simulink model "souk_dual_pipeline_krm"  (R2021a)
settings: Solver=VariableStepAuto  StartTime=0.0  StopTime=10.0  RelTol=1e-3
undefined symbols (not defined in the file): datetime, emio_enet2_tsu_timer_cmp_val_0, posixtime, signal
libraries: xbsIndex_r4 x15746, casper_library_misc x108, casper_library_delays x65, casper_library_reorder x44, xps_library x12
(part 3 of 175)

== system souk_dual_pipeline_krm/KRM4ZUxx ==

== system souk_dual_pipeline_krm/bus_expand ==
  bus_in : Inport
  reinterpret1 : xbsIndex_r4/Reinterpret  force_arith_type=on  arith_type=Unsigned  force_bin_pt=on  bin_pt=0  block_type=reinterpret
  reinterpret2 : xbsIndex_r4/Reinterpret  force_arith_type=on  arith_type=Unsigned  force_bin_pt=on  bin_pt=0  block_type=reinterpret
  slice1 : xbsIndex_r4/Slice  nbits=256  boolean_output=off  mode=Upper Bit Location + Width  bit1=-256  base1=MSB of Input  bit0=0  base0=LSB of Input  dbl_ovrd=off  block_type=slice
  slice2 : xbsIndex_r4/Slice  nbits=256  boolean_output=off  mode=Upper Bit Location + Width  bit1=0  base1=MSB of Input  bit0=0  base0=LSB of Input  dbl_ovrd=off  block_type=slice
  msb_out2 : Outport  VectorParamsAs1DForOutWhenUnconnected=off
  lsb_out1 : Outport  Port=2  VectorParamsAs1DForOutWhenUnconnected=off
  wires:
  bus_in/1 -> slice2/1, slice1/1
  slice2/1 -> reinterpret2/1
  reinterpret2/1 -> msb_out2/1
  slice1/1 -> reinterpret1/1
  reinterpret1/1 -> lsb_out1/1

== system souk_dual_pipeline_krm/bus_expand1 ==
  bus_in : Inport
  reinterpret1 : xbsIndex_r4/Reinterpret  force_arith_type=on  arith_type=Unsigned  force_bin_pt=on  bin_pt=0  block_type=reinterpret
  reinterpret2 : xbsIndex_r4/Reinterpret  force_arith_type=on  arith_type=Unsigned  force_bin_pt=on  bin_pt=0  block_type=reinterpret
  slice1 : xbsIndex_r4/Slice  nbits=256  boolean_output=off  mode=Upper Bit Location + Width  bit1=-256  base1=MSB of Input  bit0=0  base0=LSB of Input  dbl_ovrd=off  block_type=slice
  slice2 : xbsIndex_r4/Slice  nbits=256  boolean_output=off  mode=Upper Bit Location + Width  bit1=0  base1=MSB of Input  bit0=0  base0=LSB of Input  dbl_ovrd=off  block_type=slice
  msb_out2 : Outport  VectorParamsAs1DForOutWhenUnconnected=off
  lsb_out1 : Outport  Port=2  VectorParamsAs1DForOutWhenUnconnected=off
  wires:
  reinterpret1/1 -> lsb_out1/1
  slice1/1 -> reinterpret1/1
  reinterpret2/1 -> msb_out2/1
  slice2/1 -> reinterpret2/1
  bus_in/1 -> slice1/1, slice2/1

== system souk_dual_pipeline_krm/common ==
  note: flip channels and
      | put first sample in MSB
  autocorr_sync0 : Inport
  autocorr_din0 : Inport  Port=2
  autocorr_rst0 : Inport  Port=3
  autocorr_sync1 : Inport  Port=4
  autocorr_din1 : Inport  Port=5
  autocorr_rst1 : Inport  Port=6
  autocorr_sync2 : Inport  Port=7
  autocorr_din2 : Inport  Port=8
  autocorr_rst2 : Inport  Port=9
  autocorr_sync3 : Inport  Port=10
  autocorr_din3 : Inport  Port=11
  autocorr_rst3 : Inport  Port=12
  input0 : Inport  Port=13
  input1 : Inport  Port=14
  input2 : Inport  Port=15
  input3 : Inport  Port=16
  output0 : Inport  Port=17
  output1 : Inport  Port=18
  output2 : Inport  Port=19
  output3 : Inport  Port=20
  tt0 : Inport  Port=21
  tt1 : Inport  Port=22
  tt2 : Inport  Port=23
  tt3 : Inport  Port=24
  Delay{,1..29} (30 alike) : xbsIndex_r4/Delay  rst=off  infoeditControl=Selection of Reset will increase slice count due to use of real FFs and instead of SRLs  en=off  latency=1  reg_retiming=off  dbl_ovrd=off  block_type=delay
  Mux{,1..5} (6 alike) : xbsIndex_r4/Mux  inputs=4  en=off  latency=1  precision=Full  arith_type=Unsigned  n_bits=16  bin_pt=14  quantization=Truncate  overflow=Wrap  dbl_ovrd=off  block_type=mux
  adc_ss : Subsystem  mask{ram_depth_bits=9}
      mask prompts: ram_depth_bits "Ram depth (2^?)"
  autocorr : Subsystem  mask{nchan_bits=13-4, npol_bits=0}
      mask prompts: nchan_bits "Number of *SERIAL* channels (2^?)"; npol_bits "Number of pols (2^?)"
  bus_expand : Subsystem  AncestorBlock=casper_library_flow_control/bus_expand  mask(bus_expand){mode=divisions of equal size, outputNum=2, outputWidth=16*8, outputBinaryPt=0, outputArithmeticType=0, show_format=off, outputToWorkspace=off, variablePrefix=out, outputToModelAsWell=on}
      mask prompts: outputNum "Number of outputs:"; outputWidth "Output width:"; outputBinaryPt "Output binary point position:"; outputArithmeticType "Output arithmetic type (ufix=0, fix=1, bool=2):"; show_format "Print format string?"; outputToWorkspace "Output to workspace?"; variablePrefix "Variable name prefix:"; outputToModelAsWell "Output to model as well?"
      mask help:
      | Expands a 'bus' made using a bus_create or Xilinx
      | concat block.
      | The input will be divided into the specified number
      | of outputs with the specified arithmetic types.
      | Divisions are made from most significant bit.
      mask init: same as souk_dual_pipeline_krm/bus_expand
      settings: AttributesFormatString=2 outputs
      mask TypeOptions mode: divisions of equal size | divisions of arbitrary size
      mask Callback mode: %bus_expand_callback();
      mask Callback outputWidth: %bus_expand_callback();
      mask Callback outputToWorkspace: %bus_expand_callback();
  bus_expand1 : Subsystem  AncestorBlock=casper_library_flow_control/bus_expand  mask(bus_expand){mode=divisions of equal size, outputNum=2, outputWidth=16*16, outputBinaryPt=0, outputArithmeticType=0, show_format=off, outputToWorkspace=off, variablePrefix=out, outputToModelAsWell=on}
      mask prompts: outputNum "Number of outputs:"; outputWidth "Output width:"; outputBinaryPt "Output binary point position:"; outputArithmeticType "Output arithmetic type (ufix=0, fix=1, bool=2):"; show_format "Print format string?"; outputToWorkspace "Output to workspace?"; variablePrefix "Variable name prefix:"; outputToModelAsWell "Output to model as well?"
      mask help:
      | Expands a 'bus' made using a bus_create or Xilinx
      | concat block.
      | The input will be divided into the specified number
      | of outputs with the specified arithmetic types.
      | Divisions are made from most significant bit.
      mask init: same as souk_dual_pipeline_krm/bus_expand
      settings: AttributesFormatString=2 outputs
      mask TypeOptions mode: divisions of equal size | divisions of arbitrary size
      mask Callback mode: %bus_expand_callback();
      mask Callback outputWidth: %bus_expand_callback();
      mask Callback outputToWorkspace: %bus_expand_callback();
  cordic_gen : Subsystem  mask{n_cordic=1, n_parallel=8}
      mask prompts: n_cordic "Number of independent generators?"; n_parallel "Number of parallel samples?"
  dac_ss : Subsystem  mask{ram_depth_bits=9}
      mask prompts: ram_depth_bits "Ram depth (2^?)"
  iq_deinterleave : Subsystem  AncestorBlock=casper_library_flow_control/munge  mask(munge){divisions=16, div_size=16*ones(16,1), order=reshape(transpose(reshape([0:15], [2,8])), [16,1]), arith_type_out=Unsigned, bin_pt_out=0}
      mask prompts: divisions "Number of divisions"; div_size "Division size (bits)"; order "Division packing order"; arith_type_out "Output arithmetic type"; bin_pt_out "Output binary point"
      mask help: Splits an input bus into the specified number of divisions and then recombines them in the order specified (most significant division = 0,least = number divisions-1)
      mask init:
      | munge_init(gcb, ...
      |     'divisions', divisions, ...
      |     'div_size', div_size, ...
      |     'order', order, ...
      |     'arith_type_out', arith_type_out, ...
      |     'bin_pt_out', bin_pt_out);
      settings: AttributesFormatString=|
      | split:[16;16;16;16;16;16;16;16;16;16;16;16;16;16;16;16]
      | join:[0;2;4;6;8;10;12;14;1;3;5;7;9;11;13;15]
      | Unsigned [256,0]
      mask TypeOptions arith_type_out: Unsigned | Signed  (2's comp) | Floating-point
  lut_gen : Subsystem  mask{n_generator=1, n_parallel=8, n_sample_bits=13}
      mask prompts: n_generator "Number of independent generators?"; n_parallel "Number of parallel samples?"; n_sample_bits "Number of samples total (2^?)"
  munge : Subsystem  AncestorBlock=casper_library_flow_control/munge  mask(munge){divisions=32, div_size=16*ones(32,1), order=[31:-1:0], arith_type_out=Unsigned, bin_pt_out=0}
      mask prompts: divisions "Number of divisions"; div_size "Division size (bits)"; order "Division packing order"; arith_type_out "Output arithmetic type"; bin_pt_out "Output binary point"
      mask help: Splits an input bus into the specified number of divisions and then recombines them in the order specified (most significant division = 0,least = number divisions-1)
      mask init:
      | munge_init(gcb, ...
      |     'divisions', divisions, ...
      |     'div_size', div_size, ...
      |     'order', order, ...
      |     'arith_type_out', arith_type_out, ...
      |     'bin_pt_out', bin_pt_out);
      settings: AttributesFormatString=|
      | split:[16;16;16;16;16;16;16;16;16;16;16;16;16;16;16;16;16;16;16;16;16;16;16;16;16;16;16;16;16;16;16;16]
      | join:[31 30 29 28 27 26 25 24 23 22 21 20 19 18 17 16 15 14 13 12 11 10 9 8 7 6 5 4 3 2 1 0]
      | Unsigned [512,0]
      mask TypeOptions arith_type_out: Unsigned | Signed  (2's comp) | Floating-point
  sel : Subsystem  Tag=xps:sw_reg  AncestorBlock=xps_library/Memory/software_register  mask(swreg){io_dir=From Processor, io_delay=0, init_val=dec2hex(0), sample_period=1, names=reg, bitwidths=2, bin_pts=0, arith_types=0, sim_port=on, show_format=on, desc_str=""}
      mask prompts: io_dir "I/O direction"; io_delay "I/O delay"; init_val "Initial Value"; sample_period "Sample period"; names "Bitfield names [msb...lsb]"; bitwidths "Bitfield widths"; bin_pts "Bitfield binary pts"; arith_types "Bitfield types, ufix=0, fix=1, bool=2"; sim_port "Provide sim input/output?"; show_format "Print format string?"; desc_str "Description"
      mask help: A 32-bit software-accessible register. Can be divided into bitfields of varying widths and types using the fields in the block mask.
      mask init:
      | swreg_init(gcb)
      settings: AttributesFormatString=1input:uf2.0 = 2 bits
      mask TypeOptions io_dir: To Processor | From Processor
      mask Callback io_dir:
      | mask_enables = get_param(gcb, 'MaskEnables');
      | mask_names = get_param(gcb, 'MaskNames');
      | if strcmp(get_param(gcb, 'io_dir'), 'To Processor'),
      |     mask_enables{ismember(mask_names, 'sample_period')} = 'off';
      | else
      |     mask_enables{ismember(mask_names, 'sample_period')} = 'on';
      | end
      | set_param(gcb, 'MaskEnables', mask_enables);
      mask DialogControl ParameterTabVar0 Prompt: Setup
  zoom_acc : Subsystem  mask{nchan_serial_bits=10, downsample_factor=512}
      mask prompts: nchan_serial_bits "Number of serial channels (2^?)"; downsample_factor "Downsample factor?"
  zoom_fft : Subsystem
  cordic_gen_out : Outport
  lut_gen_out : Outport  Port=2
  wires:
  lut_gen/1(dout) -> lut_gen_out/1
  cordic_gen/1(dout) -> cordic_gen_out/1
  autocorr_sync0/1 -> Delay6/1
  autocorr_sync1/1 -> Delay7/1
  Delay/1 -> Mux/1
  Delay1/1 -> Mux1/1
  Delay2/1 -> Mux2/1
  zoom_fft/1(sync_out) -> zoom_acc/1(sync)
  zoom_fft/2(dout) -> zoom_acc/2(din)
  Mux2/1 -> autocorr/3(rst)
  Mux1/1 -> zoom_fft/2(din), autocorr/2(din)
  Mux/1 -> zoom_fft/1(sync), autocorr/1(sync)
  Delay6/1 -> Mux/2
  Delay7/1 -> Mux/3
  autocorr_sync2/1 -> Delay8/1
  Delay8/1 -> Mux/4
  autocorr_sync3/1 -> Delay9/1
  Delay9/1 -> Mux/5
  autocorr_din0/1 -> Delay10/1
  Delay10/1 -> Mux1/2
  autocorr_din1/1 -> Delay11/1
  Delay11/1 -> Mux1/3
  autocorr_din2/1 -> Delay12/1
  Delay12/1 -> Mux1/4
  autocorr_din3/1 -> Delay13/1
  Delay13/1 -> Mux1/5
  Delay14/1 -> Mux2/2
  Delay15/1 -> Mux2/3
  Delay16/1 -> Mux2/4
  Delay17/1 -> Mux2/5
  autocorr_rst0/1 -> Delay14/1
  autocorr_rst1/1 -> Delay15/1
  autocorr_rst2/1 -> Delay16/1
  autocorr_rst3/1 -> Delay17/1
  input3/1 -> Delay21/1
  input2/1 -> Delay20/1
  input1/1 -> Delay19/1
  input0/1 -> Delay18/1
  Delay21/1 -> Mux3/5
  Delay20/1 -> Mux3/4
  Delay19/1 -> Mux3/3
  Delay18/1 -> Mux3/2
  sel/1(in_reg) -> Delay25/1, Delay24/1, Delay22/1, Delay2/1, Delay1/1, Delay/1
  Delay22/1 -> Mux3/1
  bus_expand/1(msb_out2) -> adc_ss/1(din_i)
  bus_expand/2(lsb_out1) -> adc_ss/2(din_q)
  iq_deinterleave/1(dout) -> bus_expand/1(bus_in)
  Mux3/1 -> iq_deinterleave/1(din)
  Mux4/1 -> munge/1(din)
  Delay3/1 -> Mux4/2
  Delay4/1 -> Mux4/3
  Delay5/1 -> Mux4/4
  Delay23/1 -> Mux4/5
  output0/1 -> Delay3/1
  output1/1 -> Delay4/1
  output2/1 -> Delay5/1
  output3/1 -> Delay23/1
  Delay24/1 -> Mux4/1
  munge/1(dout) -> bus_expand1/1(bus_in)
  bus_expand1/1(msb_out2) -> dac_ss/1(din0)
  bus_expand1/2(lsb_out1) -> dac_ss/2(din1)
  tt0/1 -> Delay26/1
  tt1/1 -> Delay27/1
  tt3/1 -> Delay29/1
  tt2/1 -> Delay28/1
  Delay25/1 -> Mux5/1
  Delay26/1 -> Mux5/2
  Delay27/1 -> Mux5/3
  Delay28/1 -> Mux5/4
  Delay29/1 -> Mux5/5
  Mux5/1 -> adc_ss/3(tt), dac_ss/3(tt)

== system souk_dual_pipeline_krm/p0 ==
  note: output here has first sample in LSBs.
      | Real part in LSBs.
      | Even chans in LSBs; Odd chans in MSBs
  din_i : Inport
  din_q : Inport  Port=2
  sync_in : Inport  Port=3
  cordic_gen : Inport  Port=4
  lut_gen : Inport  Port=5
  gpio_in : Inport  Port=6
  Concat{,1..4} (5 alike) : xbsIndex_r4/Concat  num_inputs=2  dbl_ovrd=off  block_type=concat
  Constant : xbsIndex_r4/Constant  const=0  gui_display_data_type=Fixed-point  arith_type=Unsigned  n_bits=32*8  bin_pt=0  preci_type=Single  exp_width=8  frac_width=24  explicit_period=off  period=1  equ=P=C  opselect=C  inp2=PCIN>>17  opr=+  inp1=P  carry=CIN  dbl_ovrd=off  block_type=constant
  Constant1 : xbsIndex_r4/Constant  const=0  gui_display_data_type=Fixed-point  arith_type=Unsigned  n_bits=32*8  bin_pt=0  preci_type=Single  exp_width=8  frac_width=24  explicit_period=off  period=1  equ=P=C  opselect=C  inp2=PCIN>>17  opr=+  inp1=P  carry=CIN  dbl_ovrd=off  block_type=constant
  Constant2 : xbsIndex_r4/Constant  const=0  gui_display_data_type=Fixed-point  arith_type=Unsigned  n_bits=32*8  bin_pt=0  preci_type=Single  exp_width=8  frac_width=24  explicit_period=off  period=1  equ=P=C  opselect=C  inp2=PCIN>>17  opr=+  inp1=P  carry=CIN  dbl_ovrd=off  block_type=constant
  Convert : xbsIndex_r4/Convert  gui_display_data_type=Fixed-point  arith_type=Unsigned  n_bits=16  bin_pt=0  float_type=Single  exp_bits=8  fraction_bits=24  quantization=Truncate  overflow=Wrap  en=off  latency=0  pipeline=off  dbl_ovrd=off  block_type=convert
  Convert1 : xbsIndex_r4/Convert  gui_display_data_type=Fixed-point  arith_type=Unsigned  n_bits=16  bin_pt=0  float_type=Single  exp_bits=8  fraction_bits=24  quantization=Truncate  overflow=Wrap  en=off  latency=0  pipeline=off  dbl_ovrd=off  block_type=convert
  Delay : xbsIndex_r4/Delay  rst=off  infoeditControl=Selection of Reset will increase slice count due to use of real FFs and instead of SRLs  en=off  latency=1  reg_retiming=on  dbl_ovrd=off  block_type=delay
  Delay1 : xbsIndex_r4/Delay  rst=off  infoeditControl=Selection of Reset will increase slice count due to use of real FFs and instead of SRLs  en=off  latency=1  reg_retiming=on  dbl_ovrd=off  block_type=delay
  Delay2 : xbsIndex_r4/Delay  rst=off  infoeditControl=Selection of Reset will increase slice count due to use of real FFs and instead of SRLs  en=off  latency=1  reg_retiming=on  dbl_ovrd=off  block_type=delay
  Mux : xbsIndex_r4/Mux  inputs=2  en=off  latency=1  precision=Full  arith_type=Unsigned  n_bits=16  bin_pt=14  quantization=Truncate  overflow=Wrap  dbl_ovrd=off  block_type=mux
  Terminator{,1,3..4} (4 alike) : Terminator
  acc0 : Subsystem  mask{nchan_serial_bits=11, nwindow_bits=11}
      mask prompts: nchan_serial_bits "Number of serial channels (2^?)"; nwindow_bits "Window points (2^?)"
  bus_addsub : Subsystem  AncestorBlock=casper_library_bus/bus_addsub  mask(bus_addsub){opmode=0, n_bits_a=ones(8,1) * 16, bin_pt_a=ones(8,1) * 15, type_a=1, n_bits_b=ones(8,1) * 16, bin_pt_b=ones(8,1) * 15, type_b=1, cmplx=on, misc=off, async=off, floating_point=off, float_type=single, exp_width=6, frac_width=19, n_bits_out=ones(8,1) * 16, bin_pt_out=ones(8,1) * 15, type_out=1, quantization=0, overflow=1, add_implementation=fabric core, csp_latency=1, pipeline_en=off, pipeline_latency=0}
      mask prompts: opmode "mode (Addition=0, Subtraction=1)"; n_bits_a "a input bit widths"; bin_pt_a "a input binary points"; type_a "a input type (Unsigned=0, Signed=1)"; n_bits_b "b input bit widths"; bin_pt_b "b input binary points"; type_b "b input type (Unsigned=0, Signed=1)"; cmplx "complex"; misc "misc support"; async "asynchronous operation"; floating_point "floating point"; exp_width "exponent width"; frac_width "fraction width"; n_bits_out "output bit widths"; bin_pt_out "output binary points"; type_out "output type (Unsigned=0, Signed=1)"; quantization "quantization strategy (Truncate=0, Round  (unbiased: +/- Inf)=1)"; overflow "overflow strategy (Wrap=0, Saturate=1, Flag as error=2)"; add_implementation "adder implementation"; csp_latency "latency"; pipeline_en "pipeline enable"; pipeline_latency "pipeline latency"
      mask help: Add/subtract components of two busses
      mask init:
      | bus_addsub_init(gcb, ...
      |     'opmode', opmode, ...
      |     'n_bits_a', n_bits_a, ...
      |     'bin_pt_a', bin_pt_a, ...
      |     'type_a', type_a, ...
      |     'n_bits_b', n_bits_b, ...
      |     'bin_pt_b', bin_pt_b, ...
      |     'type_b', type_b, ...
      |     'n_bits_out', n_bits_out, ...
      |     'bin_pt_out', bin_pt_out, ...
      |     'floating_point', floating_point, ...
      |     'float_type', float_type, ...
      |     'exp_width', exp_width, ...
      |     'frac_width', frac_width, ...
      |     'type_out', type_out, ...
      |     'overflow', overflow, ...        
      |     'quantization', quantization, ...
      |     'add_implementation', add_implementation, ...
      |     'csp_latency', csp_latency, ...
      |     'pipeline_en', pipeline_en, ...
      |     'pipeline_latency', pipeline_latency,...
      |     'cmplx', cmplx, ...
      |     'misc', misc, ...
      |     'async', async);
      mask Callback floating_point:
      | onoff = get_param(gcb, 'floating_point');
      | if strcmp(onoff,'on')
      |     enable_fixpt = 'off';
      |     set_param_state(gcb, 'float_type', 'on')
      | 
      |     f_type = get_param(gcb, 'float_type');
      |     if strcmp(f_type,'custom')
      |         set_param_state(gcb, 'exp_width', 'on')
      |         set_param_state(gcb, 'frac_width', 'on')
      |     else
      |         set_param_state(gcb, 'exp_width', 'off')
      |         set_param_state(gcb, 'frac_width', 'off')
      |     end
      | 
      | 
      | else
      |     enable_fixpt = 'on';
      |     set_param_state(gcb, 'float_type', 'off')
      |     set_param_state(gcb, 'exp_width', 'off')
      |     set_param_state(gcb, 'frac_width', 'off')
      | end
      | 
      | set_param_state(gcb, 'n_bits_a', enable_fixpt)
      | set_param_state(gcb, 'bin_pt_a', enable_fixpt)
      | set_param_state(gcb, 'type_a', enable_fixpt)
      | set_param_state(gcb, 'n_bits_b', enable_fixpt)
      | set_param_state(gcb, 'bin_pt_b', enable_fixpt)
      | set_param_state(gcb, 'type_b', enable_fixpt)
      | 
      | set_param_state(gcb, 'n_bits_out', enable_fixpt)
      | set_param_state(gcb, 'bin_pt_out', enable_fixpt)
      | set_param_state(gcb, 'type_out', enable_fixpt)
      | set_param_state(gcb, 'quantization', enable_fixpt)
      | set_param_state(gcb, 'overflow', enable_fixpt)
      mask TypeOptions float_type: single | custom
      mask Callback float_type:
      | f_type = get_param(gcb, 'float_type');
      | if strcmp(f_type,'custom')
      |     set_param_state(gcb, 'exp_width', 'on')
      |     set_param_state(gcb, 'frac_width', 'on')
      | else
      |     set_param_state(gcb, 'exp_width', 'off')
      |     set_param_state(gcb, 'frac_width', 'off')
      | end
      mask TypeOptions add_implementation: behavioral HDL | fabric core | DSP48 core
  bus_expand : Subsystem  AncestorBlock=casper_library_flow_control/bus_expand  mask(bus_expand){mode=divisions of equal size, outputNum=2, outputWidth=256, outputBinaryPt=0, outputArithmeticType=0, show_format=off, outputToWorkspace=off, variablePrefix=out, outputToModelAsWell=on}
      mask prompts: outputNum "Number of outputs:"; outputWidth "Output width:"; outputBinaryPt "Output binary point position:"; outputArithmeticType "Output arithmetic type (ufix=0, fix=1, bool=2):"; show_format "Print format string?"; outputToWorkspace "Output to workspace?"; variablePrefix "Variable name prefix:"; outputToModelAsWell "Output to model as well?"
      mask help:
      | Expands a 'bus' made using a bus_create or Xilinx
      | concat block.
      | The input will be divided into the specified number
      | of outputs with the specified arithmetic types.
      | Divisions are made from most significant bit.
      mask init: same as souk_dual_pipeline_krm/bus_expand
      settings: AttributesFormatString=2 outputs
      mask TypeOptions mode: divisions of equal size | divisions of arbitrary size
      mask Callback mode: %bus_expand_callback();
      mask Callback outputWidth: %bus_expand_callback();
      mask Callback outputToWorkspace: %bus_expand_callback();
  chan_select : Subsystem  mask{serial_chan_bits=9, parallel_chan_bits=4, parallel_samp_bits=2}
      mask prompts: serial_chan_bits "Number of serial channels (2^?)"; parallel_chan_bits "Number of parallel channels (2^?)"; parallel_samp_bits "Number of parallel samples out (2^?)"
  input : Subsystem
  mix : Subsystem  mask{serial_chan_bits=11, phase_slot_bits=12, lo_slot_bits=2}
      mask prompts: serial_chan_bits "Number of serial channels (2^?)"; phase_slot_bits "Number of phase switching slots (2^?)"; lo_slot_bits "Number of LO slots (2?)"
  outdelay : Subsystem
  output : Subsystem
  pfb : Subsystem
  pfbtvg : Subsystem  mask{serial_chan_bits=9, parallel_chan_bits=4}
      mask prompts: serial_chan_bits "Serial channels (2^?)"; parallel_chan_bits "Parallel channels (2^?)"
  psb : Subsystem
  pulse_ext : Subsystem  AncestorBlock=casper_library_misc/pulse_ext  mask(pulse_ext){pulse_len=2^25}
      mask prompts: pulse_len "Length of Pulse"
      mask help:
      | Extends a boolean signal to be high for the specified number of clocks after
      | the last high input.
      mask init:
      | bits = ceil(log2(pulse_len+1));
      mask Help: eval('xlWeb(''http://casper.berkeley.edu/wiki/Pulse_ext'')')
  sync : Subsystem  mask{sync_lsb_bits=1, sync_period=307200000}
      mask prompts: sync_lsb_bits "Allowed sync granularity (2^?)"; sync_period "Expected_sync_period"
  synth_input_reorder : Subsystem  mask{serial_chan_bits=9, parallel_chan_bits=4, parallel_samp_bits=2}
      mask prompts: serial_chan_bits "Number of serial channels out (2^?)"; parallel_chan_bits "Number of parallel channels out (2^?)"; parallel_samp_bits "Number of parallel samples in (2^?)"
  synth_input_reorder1 : Subsystem  Commented=on  mask{serial_chan_bits=9, parallel_chan_bits=2}
      mask prompts: serial_chan_bits "Number of serial channels (2^?)"; parallel_chan_bits "Number of parallel channels (2^?)"
  synth_input_reorder3 : Subsystem  Commented=on  mask{serial_chan_bits=9, parallel_chan_bits=4, parallel_samp_bits=2}
      mask prompts: serial_chan_bits "Number of serial channels out (2^?)"; parallel_chan_bits "Number of parallel channels out (2^?)"; parallel_samp_bits "Number of parallel samples in (2^?)"
  use_dual_dac : Subsystem  Tag=xps:sw_reg  AncestorBlock=xps_library/Memory/software_register  mask(swreg){io_dir=From Processor, io_delay=0, init_val=dec2hex(0), sample_period=1, names=reg, bitwidths=1, bin_pts=0, arith_types=0, sim_port=on, show_format=on, desc_str=""}
      mask prompts: io_dir "I/O direction"; io_delay "I/O delay"; init_val "Initial Value"; sample_period "Sample period"; names "Bitfield names [msb...lsb]"; bitwidths "Bitfield widths"; bin_pts "Bitfield binary pts"; arith_types "Bitfield types, ufix=0, fix=1, bool=2"; sim_port "Provide sim input/output?"; show_format "Print format string?"; desc_str "Description"
      mask help: A 32-bit software-accessible register. Can be divided into bitfields of varying widths and types using the fields in the block mask.
      mask init:
      | swreg_init(gcb)
      settings: AttributesFormatString=1input:uf1.0 = 1 bits
      mask TypeOptions io_dir: To Processor | From Processor
      mask Callback io_dir:
      | mask_enables = get_param(gcb, 'MaskEnables');
      | mask_names = get_param(gcb, 'MaskNames');
      | if strcmp(get_param(gcb, 'io_dir'), 'To Processor'),
      |     mask_enables{ismember(mask_names, 'sample_period')} = 'off';
      | else
      |     mask_enables{ismember(mask_names, 'sample_period')} = 'on';
      | end
      | set_param(gcb, 'MaskEnables', mask_enables);
      mask DialogControl ParameterTabVar0 Prompt: Setup
  dout : Outport
  pps_led : Outport  Port=2
  ac_sync : Outport  Port=3
  ac_data : Outport  Port=4
  ac_rst : Outport  Port=5
  input_out : Outport  Port=6
  new_acc0 : Outport  Port=7
  tt_int_out : Outport  Port=8
  wires:
  chan_select/1(sync_out) -> mix/1(sync_rx)
  [mrst] -> mix/4(rst)
  input/2(dout) -> input_out/1, pfb/2(din)
  sync/1(arm_noise) -> Terminator/1
  chan_select/2(dout0) -> mix/2(din)
  din_i/1 -> Delay1/1
  sync/7(tt_int_out) -> tt_int_out/1
  sync/8(err_out) -> Terminator3/1
  mix/5(dout) -> acc0/3(din)
  sync/6(timed_sync) -> [sync_gen]
  pfb/2(dout) -> pfbtvg/2(din)
  din_q/1 -> Delay/1
  pfb/1(sync_out) -> pfbtvg/1(sync)
  mix/4(tt_out) -> acc0/2(tt)
  pfbtvg/1(sync_out) -> ac_sync/1, chan_select/1(sync)
  sync/5(mrst) -> [mrst]
  input/1(sync_out) -> pfb/1(sync)
  sync_in/1 -> sync/1(sync_in)
  sync/3(ext_sync) -> pulse_ext/1(in)
  pulse_ext/1(out) -> pps_led/1
  output/2(dout) -> outdelay/1(din)
  [mrst] -> ac_rst/1
  pfbtvg/2(dout) -> ac_data/1, chan_select/2(din)
  synth_input_reorder/1(sync_out) -> psb/1(sync)
  Concat/1 -> output/4(in_psb)
  psb/2(dout0) -> Concat/1
  psb/3(dout1) -> Concat/2
  Concat1/1 -> output/2(in_cordic)
  Concat2/1 -> output/3(in_lut)
  cordic_gen/1 -> Concat1/1
  lut_gen/1 -> Concat2/1
  Constant/1 -> Concat2/2
  Constant1/1 -> Concat1/2
  bus_expand/1(msb_out2) -> bus_addsub/1(a)
  bus_expand/2(lsb_out1) -> bus_addsub/2(b)
  bus_addsub/1(dout) -> Concat3/2, input/4(dac)
  outdelay/1(dout) -> Mux/3, bus_expand/1(bus_in)
  synth_input_reorder/2(dout0) -> psb/2(din0)
  synth_input_reorder/3(dout1) -> psb/3(din1)
  use_dual_dac/1(in_reg) -> Mux/1
  Mux/1 -> dout/1
  Concat3/1 -> Mux/2
  Constant2/1 -> Concat3/1
  mix/6(lo_out) -> synth_input_reorder/2(din)
  mix/7(lo_sync_out) -> synth_input_reorder/1(sync)
  acc0/1(new_acc_out) -> new_acc0/1
  gpio_in/1 -> [gpio]
  [gpio] -> acc0/4(gpio)
  [sync_gen] -> mix/3(sync_tx)
  psb/1(sync_out) -> output/1(sync)
  Delay/1 -> input/3(din_q)
  Delay1/1 -> input/2(din_i)
  Delay2/1 -> input/1(sync)
  [sync_gen_delayed] -> Delay2/1
  sync/9(drift) -> [drift]
  [drift] -> acc0/5(tt_drift)
  [mrst] -> synth_input_reorder/3(rst)
  sync/4(sync_out) -> Terminator1/1
  sync/10(tt_timed_sync) -> [sync_time]
  sync/2(tt_sync) -> Terminator4/1
  mix/2(sync_to_rx) -> [sync_gen_delayed]
  [sync_time] -> mix/5(tt)
  mix/3(new_acc_out) -> acc0/1(new_acc)
  mix/9(slot_out) -> Convert1/1
  mix/8(buf_out) -> Convert/1
  Convert1/1 -> Concat4/2
  Convert/1 -> Concat4/1
  Concat4/1 -> acc0/6(buf_id)

== system souk_dual_pipeline_krm/p1 ==
  note: output here has first sample in LSBs.
      | Real part in LSBs.
      | Even chans in LSBs; Odd chans in MSBs
  din_i : Inport
  din_q : Inport  Port=2
  sync_in : Inport  Port=3
  cordic_gen : Inport  Port=4
  lut_gen : Inport  Port=5
  gpio_in : Inport  Port=6
  Concat{,1..4} (5 alike) : xbsIndex_r4/Concat  num_inputs=2  dbl_ovrd=off  block_type=concat
  Constant : xbsIndex_r4/Constant  const=0  gui_display_data_type=Fixed-point  arith_type=Unsigned  n_bits=32*8  bin_pt=0  preci_type=Single  exp_width=8  frac_width=24  explicit_period=off  period=1  equ=P=C  opselect=C  inp2=PCIN>>17  opr=+  inp1=P  carry=CIN  dbl_ovrd=off  block_type=constant
  Constant1 : xbsIndex_r4/Constant  const=0  gui_display_data_type=Fixed-point  arith_type=Unsigned  n_bits=32*8  bin_pt=0  preci_type=Single  exp_width=8  frac_width=24  explicit_period=off  period=1  equ=P=C  opselect=C  inp2=PCIN>>17  opr=+  inp1=P  carry=CIN  dbl_ovrd=off  block_type=constant
  Constant2 : xbsIndex_r4/Constant  const=0  gui_display_data_type=Fixed-point  arith_type=Unsigned  n_bits=32*8  bin_pt=0  preci_type=Single  exp_width=8  frac_width=24  explicit_period=off  period=1  equ=P=C  opselect=C  inp2=PCIN>>17  opr=+  inp1=P  carry=CIN  dbl_ovrd=off  block_type=constant
  Convert : xbsIndex_r4/Convert  gui_display_data_type=Fixed-point  arith_type=Unsigned  n_bits=16  bin_pt=0  float_type=Single  exp_bits=8  fraction_bits=24  quantization=Truncate  overflow=Wrap  en=off  latency=0  pipeline=off  dbl_ovrd=off  block_type=convert
  Convert1 : xbsIndex_r4/Convert  gui_display_data_type=Fixed-point  arith_type=Unsigned  n_bits=16  bin_pt=0  float_type=Single  exp_bits=8  fraction_bits=24  quantization=Truncate  overflow=Wrap  en=off  latency=0  pipeline=off  dbl_ovrd=off  block_type=convert
  Delay : xbsIndex_r4/Delay  rst=off  infoeditControl=Selection of Reset will increase slice count due to use of real FFs and instead of SRLs  en=off  latency=1  reg_retiming=on  dbl_ovrd=off  block_type=delay
  Delay1 : xbsIndex_r4/Delay  rst=off  infoeditControl=Selection of Reset will increase slice count due to use of real FFs and instead of SRLs  en=off  latency=1  reg_retiming=on  dbl_ovrd=off  block_type=delay
  Delay2 : xbsIndex_r4/Delay  rst=off  infoeditControl=Selection of Reset will increase slice count due to use of real FFs and instead of SRLs  en=off  latency=1  reg_retiming=on  dbl_ovrd=off  block_type=delay
  Mux : xbsIndex_r4/Mux  inputs=2  en=off  latency=1  precision=Full  arith_type=Unsigned  n_bits=16  bin_pt=14  quantization=Truncate  overflow=Wrap  dbl_ovrd=off  block_type=mux
  Terminator{,1,3..4} (4 alike) : Terminator
  acc0 : Subsystem  mask{nchan_serial_bits=11, nwindow_bits=11}
      mask prompts: nchan_serial_bits "Number of serial channels (2^?)"; nwindow_bits "Window points (2^?)"
  bus_addsub : Subsystem  AncestorBlock=casper_library_bus/bus_addsub  mask(bus_addsub){opmode=0, n_bits_a=ones(8,1) * 16, bin_pt_a=ones(8,1) * 15, type_a=1, n_bits_b=ones(8,1) * 16, bin_pt_b=ones(8,1) * 15, type_b=1, cmplx=on, misc=off, async=off, floating_point=off, float_type=single, exp_width=6, frac_width=19, n_bits_out=ones(8,1) * 16, bin_pt_out=ones(8,1) * 15, type_out=1, quantization=0, overflow=1, add_implementation=fabric core, csp_latency=1, pipeline_en=off, pipeline_latency=0}
      mask prompts: opmode "mode (Addition=0, Subtraction=1)"; n_bits_a "a input bit widths"; bin_pt_a "a input binary points"; type_a "a input type (Unsigned=0, Signed=1)"; n_bits_b "b input bit widths"; bin_pt_b "b input binary points"; type_b "b input type (Unsigned=0, Signed=1)"; cmplx "complex"; misc "misc support"; async "asynchronous operation"; floating_point "floating point"; exp_width "exponent width"; frac_width "fraction width"; n_bits_out "output bit widths"; bin_pt_out "output binary points"; type_out "output type (Unsigned=0, Signed=1)"; quantization "quantization strategy (Truncate=0, Round  (unbiased: +/- Inf)=1)"; overflow "overflow strategy (Wrap=0, Saturate=1, Flag as error=2)"; add_implementation "adder implementation"; csp_latency "latency"; pipeline_en "pipeline enable"; pipeline_latency "pipeline latency"
      mask help: Add/subtract components of two busses
      mask init: same as souk_dual_pipeline_krm/p0/bus_addsub
      mask Callback floating_point:
      | onoff = get_param(gcb, 'floating_point');
      | if strcmp(onoff,'on')
      |     enable_fixpt = 'off';
      |     set_param_state(gcb, 'float_type', 'on')
      | 
      |     f_type = get_param(gcb, 'float_type');
      |     if strcmp(f_type,'custom')
      |         set_param_state(gcb, 'exp_width', 'on')
      |         set_param_state(gcb, 'frac_width', 'on')
      |     else
      |         set_param_state(gcb, 'exp_width', 'off')
      |         set_param_state(gcb, 'frac_width', 'off')
      |     end
      | 
      | 
      | else
      |     enable_fixpt = 'on';
      |     set_param_state(gcb, 'float_type', 'off')
      |     set_param_state(gcb, 'exp_width', 'off')
      |     set_param_state(gcb, 'frac_width', 'off')
      | end
      | 
      | set_param_state(gcb, 'n_bits_a', enable_fixpt)
      | set_param_state(gcb, 'bin_pt_a', enable_fixpt)
      | set_param_state(gcb, 'type_a', enable_fixpt)
      | set_param_state(gcb, 'n_bits_b', enable_fixpt)
      | set_param_state(gcb, 'bin_pt_b', enable_fixpt)
      | set_param_state(gcb, 'type_b', enable_fixpt)
      | 
      | set_param_state(gcb, 'n_bits_out', enable_fixpt)
      | set_param_state(gcb, 'bin_pt_out', enable_fixpt)
      | set_param_state(gcb, 'type_out', enable_fixpt)
      | set_param_state(gcb, 'quantization', enable_fixpt)
      | set_param_state(gcb, 'overflow', enable_fixpt)
      mask TypeOptions float_type: single | custom
      mask Callback float_type:
      | f_type = get_param(gcb, 'float_type');
      | if strcmp(f_type,'custom')
      |     set_param_state(gcb, 'exp_width', 'on')
      |     set_param_state(gcb, 'frac_width', 'on')
      | else
      |     set_param_state(gcb, 'exp_width', 'off')
      |     set_param_state(gcb, 'frac_width', 'off')
      | end
      mask TypeOptions add_implementation: behavioral HDL | fabric core | DSP48 core
  bus_expand : Subsystem  AncestorBlock=casper_library_flow_control/bus_expand  mask(bus_expand){mode=divisions of equal size, outputNum=2, outputWidth=256, outputBinaryPt=0, outputArithmeticType=0, show_format=off, outputToWorkspace=off, variablePrefix=out, outputToModelAsWell=on}
      mask prompts: outputNum "Number of outputs:"; outputWidth "Output width:"; outputBinaryPt "Output binary point position:"; outputArithmeticType "Output arithmetic type (ufix=0, fix=1, bool=2):"; show_format "Print format string?"; outputToWorkspace "Output to workspace?"; variablePrefix "Variable name prefix:"; outputToModelAsWell "Output to model as well?"
      mask help:
      | Expands a 'bus' made using a bus_create or Xilinx
      | concat block.
      | The input will be divided into the specified number
      | of outputs with the specified arithmetic types.
      | Divisions are made from most significant bit.
      mask init: same as souk_dual_pipeline_krm/bus_expand
      settings: AttributesFormatString=2 outputs
      mask TypeOptions mode: divisions of equal size | divisions of arbitrary size
      mask Callback mode: %bus_expand_callback();
      mask Callback outputWidth: %bus_expand_callback();
      mask Callback outputToWorkspace: %bus_expand_callback();
  chan_select : Subsystem  mask{serial_chan_bits=9, parallel_chan_bits=4, parallel_samp_bits=2}
      mask prompts: serial_chan_bits "Number of serial channels (2^?)"; parallel_chan_bits "Number of parallel channels (2^?)"; parallel_samp_bits "Number of parallel samples out (2^?)"
  input : Subsystem
  mix : Subsystem  mask{serial_chan_bits=11, phase_slot_bits=12, lo_slot_bits=2}
      mask prompts: serial_chan_bits "Number of serial channels (2^?)"; phase_slot_bits "Number of phase switching slots (2^?)"; lo_slot_bits "Number of LO slots (2?)"
  outdelay : Subsystem
  output : Subsystem
  pfb : Subsystem
  pfbtvg : Subsystem  mask{serial_chan_bits=9, parallel_chan_bits=4}
      mask prompts: serial_chan_bits "Serial channels (2^?)"; parallel_chan_bits "Parallel channels (2^?)"
  psb : Subsystem
  pulse_ext : Subsystem  AncestorBlock=casper_library_misc/pulse_ext  mask(pulse_ext){pulse_len=2^25}
      mask prompts: pulse_len "Length of Pulse"
      mask help:
      | Extends a boolean signal to be high for the specified number of clocks after
      | the last high input.
      mask init:
      | bits = ceil(log2(pulse_len+1));
      mask Help: eval('xlWeb(''http://casper.berkeley.edu/wiki/Pulse_ext'')')
  sync : Subsystem  mask{sync_lsb_bits=1, sync_period=307200000}
      mask prompts: sync_lsb_bits "Allowed sync granularity (2^?)"; sync_period "Expected_sync_period"
  synth_input_reorder : Subsystem  mask{serial_chan_bits=9, parallel_chan_bits=4, parallel_samp_bits=2}
      mask prompts: serial_chan_bits "Number of serial channels out (2^?)"; parallel_chan_bits "Number of parallel channels out (2^?)"; parallel_samp_bits "Number of parallel samples in (2^?)"
  synth_input_reorder1 : Subsystem  Commented=on  mask{serial_chan_bits=9, parallel_chan_bits=2}
      mask prompts: serial_chan_bits "Number of serial channels (2^?)"; parallel_chan_bits "Number of parallel channels (2^?)"
  synth_input_reorder3 : Subsystem  Commented=on  mask{serial_chan_bits=9, parallel_chan_bits=4, parallel_samp_bits=2}
      mask prompts: serial_chan_bits "Number of serial channels out (2^?)"; parallel_chan_bits "Number of parallel channels out (2^?)"; parallel_samp_bits "Number of parallel samples in (2^?)"
  use_dual_dac : Subsystem  Tag=xps:sw_reg  AncestorBlock=xps_library/Memory/software_register  mask(swreg){io_dir=From Processor, io_delay=0, init_val=dec2hex(0), sample_period=1, names=reg, bitwidths=1, bin_pts=0, arith_types=0, sim_port=on, show_format=on, desc_str=""}
      mask prompts: io_dir "I/O direction"; io_delay "I/O delay"; init_val "Initial Value"; sample_period "Sample period"; names "Bitfield names [msb...lsb]"; bitwidths "Bitfield widths"; bin_pts "Bitfield binary pts"; arith_types "Bitfield types, ufix=0, fix=1, bool=2"; sim_port "Provide sim input/output?"; show_format "Print format string?"; desc_str "Description"
      mask help: A 32-bit software-accessible register. Can be divided into bitfields of varying widths and types using the fields in the block mask.
      mask init:
      | swreg_init(gcb)
      settings: AttributesFormatString=1input:uf1.0 = 1 bits
      mask TypeOptions io_dir: To Processor | From Processor
      mask Callback io_dir:
      | mask_enables = get_param(gcb, 'MaskEnables');
      | mask_names = get_param(gcb, 'MaskNames');
      | if strcmp(get_param(gcb, 'io_dir'), 'To Processor'),
      |     mask_enables{ismember(mask_names, 'sample_period')} = 'off';
      | else
      |     mask_enables{ismember(mask_names, 'sample_period')} = 'on';
      | end
      | set_param(gcb, 'MaskEnables', mask_enables);
      mask DialogControl ParameterTabVar0 Prompt: Setup
  dout : Outport
  pps_led : Outport  Port=2
  ac_sync : Outport  Port=3
  ac_data : Outport  Port=4
  ac_rst : Outport  Port=5
  input_out : Outport  Port=6
  new_acc0 : Outport  Port=7
  tt_int_out : Outport  Port=8
  wires:
  Concat4/1 -> acc0/6(buf_id)
  Convert/1 -> Concat4/1
  Convert1/1 -> Concat4/2
  mix/8(buf_out) -> Convert/1
  mix/9(slot_out) -> Convert1/1
  mix/3(new_acc_out) -> acc0/1(new_acc)
  [sync_time] -> mix/5(tt)
  mix/2(sync_to_rx) -> [sync_gen_delayed]
  sync/2(tt_sync) -> Terminator4/1
  sync/10(tt_timed_sync) -> [sync_time]
  sync/4(sync_out) -> Terminator1/1
  [mrst] -> synth_input_reorder/3(rst)
  [drift] -> acc0/5(tt_drift)
  sync/9(drift) -> [drift]
  [sync_gen_delayed] -> Delay2/1
  Delay2/1 -> input/1(sync)
  Delay1/1 -> input/2(din_i)
  Delay/1 -> input/3(din_q)
  psb/1(sync_out) -> output/1(sync)
  [sync_gen] -> mix/3(sync_tx)
  [gpio] -> acc0/4(gpio)
  gpio_in/1 -> [gpio]
  acc0/1(new_acc_out) -> new_acc0/1
  mix/7(lo_sync_out) -> synth_input_reorder/1(sync)
  mix/6(lo_out) -> synth_input_reorder/2(din)
  Constant2/1 -> Concat3/1
  Concat3/1 -> Mux/2
  Mux/1 -> dout/1
  use_dual_dac/1(in_reg) -> Mux/1
  synth_input_reorder/3(dout1) -> psb/3(din1)
  synth_input_reorder/2(dout0) -> psb/2(din0)
  outdelay/1(dout) -> bus_expand/1(bus_in), Mux/3
  bus_addsub/1(dout) -> input/4(dac), Concat3/2
  bus_expand/2(lsb_out1) -> bus_addsub/2(b)
  bus_expand/1(msb_out2) -> bus_addsub/1(a)
  Constant1/1 -> Concat1/2
  Constant/1 -> Concat2/2
  lut_gen/1 -> Concat2/1
  cordic_gen/1 -> Concat1/1
  Concat2/1 -> output/3(in_lut)
  Concat1/1 -> output/2(in_cordic)
  psb/3(dout1) -> Concat/2
  psb/2(dout0) -> Concat/1
  Concat/1 -> output/4(in_psb)
  synth_input_reorder/1(sync_out) -> psb/1(sync)
  pfbtvg/2(dout) -> chan_select/2(din), ac_data/1
  [mrst] -> ac_rst/1
  output/2(dout) -> outdelay/1(din)
  pulse_ext/1(out) -> pps_led/1
  sync/3(ext_sync) -> pulse_ext/1(in)
  sync_in/1 -> sync/1(sync_in)
  input/1(sync_out) -> pfb/1(sync)
  sync/5(mrst) -> [mrst]
  pfbtvg/1(sync_out) -> chan_select/1(sync), ac_sync/1
  mix/4(tt_out) -> acc0/2(tt)
  pfb/1(sync_out) -> pfbtvg/1(sync)
  din_q/1 -> Delay/1
  pfb/2(dout) -> pfbtvg/2(din)
  sync/6(timed_sync) -> [sync_gen]
  mix/5(dout) -> acc0/3(din)
  sync/8(err_out) -> Terminator3/1
  sync/7(tt_int_out) -> tt_int_out/1
  din_i/1 -> Delay1/1
  chan_select/2(dout0) -> mix/2(din)
  sync/1(arm_noise) -> Terminator/1
  input/2(dout) -> pfb/2(din), input_out/1
  [mrst] -> mix/4(rst)
  chan_select/1(sync_out) -> mix/1(sync_rx)

== system souk_dual_pipeline_krm/pulse_ext ==
  in : Inport
  Constant5 : xbsIndex_r4/Constant  const=pulse_len  gui_display_data_type=Fixed-point  arith_type=Unsigned  n_bits=bits  bin_pt=0  preci_type=Single  exp_width=8  frac_width=24  explicit_period=off  period=1  equ=P=C  opselect=C  inp2=PCIN>>17  opr=+  inp1=P  carry=CIN  dbl_ovrd=off  block_type=constant
      settings: block_version=9.1.01
  Counter3 : xbsIndex_r4/Counter  cnt_type=Free Running  cnt_to=1023  operation=Up  start_count=0  cnt_by_val=1  arith_type=Unsigned  n_bits=bits  bin_pt=0  load_pin=off  rst=on  en=on  explicit_period=on  period=1  use_behavioral_HDL=off  implementation=Fabric  use_rpm=on  dbl_ovrd=off  block_type=counter
      settings: xl_area=[0, 0, 0, 0, 0, 0, 0]  block_version=9.1.01
  Relational5 : xbsIndex_r4/Relational  mode=a!=b  op_type=Bool  en=off  latency=0  dbl_ovrd=off  block_type=relational
      settings: xl_area=[0, 0, 0, 0, 0, 0, 0]  block_version=9.1.01
  posedge : Subsystem  AncestorBlock=casper_library_misc/edge_detect  mask(edge_detect){edge=Rising, polarity=Active High, x_in=[0 0.08 0.08 0.16 0.16 0.24 0.24 0.32 0.32 0.4], y_in=[-1 -1  1  1  1  1  1  1  1  1], x_out=[0.6 0.68 0.68 0.76 0.76 0.84 0.84 0.92 0.92 1], y_out=[-1 -1  1  1 -1 -1 -1 -1 -1 -1]}
      mask prompts: edge "Edge Type"; polarity "Output Polarity"; x_in "Input X Positions"; y_in "Input Y Positions"; x_out "Output X Positions"; y_out "Output Y Positions"
      mask help: Output is active for one-cycle after each edge of the specified type (i.e. rising, falling or both).
      mask init:
      | edge_detect_init(gcb,...
      |     'edge',edge,...
      |     'polarity',polarity,...
      |     'x_in',x_in,...
      |     'x_out',x_out,...
      |     'y_in',y_in,...
      |     'y_out',y_out);
      | 
      | x_in_num=str2num(getfield(getfield(get_param(gcb,'UserData'),'parameters'),'x_in'));
      | x_out_num=str2num(getfield(getfield(get_param(gcb,'UserData'),'parameters'),'x_out'));
      | y_in_num=str2num(getfield(getfield(get_param(gcb,'UserData'),'parameters'),'y_in'));
      | y_out_num=str2num(getfield(getfield(get_param(gcb,'UserData'),'parameters'),'y_out'));
      settings: AttributesFormatString=|
      | rising edges
      | active high
      mask Help: Output is active for one-cycle after each edge of the specified type (i.e. rising, falling, or both).  Latency is zero.
      mask TypeOptions edge: Rising | Falling | Both
      mask TypeOptions polarity: Active High | Active Low
      mask Display:
      | plot(x_in_num,0.5+y_in_num*0.2);
      | plot(x_out_num,0.5+y_out_num*0.2);
  out : Outport  VectorParamsAs1DForOutWhenUnconnected=off
  wires:
  Counter3/1 -> Relational5/1
  Constant5/1 -> Relational5/2
  Relational5/1 -> Counter3/2, out/1
  in/1 -> posedge/1(in)
  posedge/1(out) -> Counter3/1

== system souk_dual_pipeline_krm/pulse_ext1 ==
  in : Inport
  Constant5 : xbsIndex_r4/Constant  const=pulse_len  gui_display_data_type=Fixed-point  arith_type=Unsigned  n_bits=bits  bin_pt=0  preci_type=Single  exp_width=8  frac_width=24  explicit_period=off  period=1  equ=P=C  opselect=C  inp2=PCIN>>17  opr=+  inp1=P  carry=CIN  dbl_ovrd=off  block_type=constant
      settings: block_version=9.1.01
  Counter3 : xbsIndex_r4/Counter  cnt_type=Free Running  cnt_to=1023  operation=Up  start_count=0  cnt_by_val=1  arith_type=Unsigned  n_bits=bits  bin_pt=0  load_pin=off  rst=on  en=on  explicit_period=on  period=1  use_behavioral_HDL=off  implementation=Fabric  use_rpm=on  dbl_ovrd=off  block_type=counter
      settings: xl_area=[0, 0, 0, 0, 0, 0, 0]  block_version=9.1.01
  Relational5 : xbsIndex_r4/Relational  mode=a!=b  op_type=Bool  en=off  latency=0  dbl_ovrd=off  block_type=relational
      settings: xl_area=[0, 0, 0, 0, 0, 0, 0]  block_version=9.1.01
  posedge : Subsystem  AncestorBlock=casper_library_misc/edge_detect  mask(edge_detect){edge=Rising, polarity=Active High, x_in=[0 0.08 0.08 0.16 0.16 0.24 0.24 0.32 0.32 0.4], y_in=[-1 -1  1  1  1  1  1  1  1  1], x_out=[0.6 0.68 0.68 0.76 0.76 0.84 0.84 0.92 0.92 1], y_out=[-1 -1  1  1 -1 -1 -1 -1 -1 -1]}
      mask prompts: edge "Edge Type"; polarity "Output Polarity"; x_in "Input X Positions"; y_in "Input Y Positions"; x_out "Output X Positions"; y_out "Output Y Positions"
      mask help: Output is active for one-cycle after each edge of the specified type (i.e. rising, falling or both).
      mask init: same as souk_dual_pipeline_krm/pulse_ext/posedge
      settings: AttributesFormatString=|
      | rising edges
      | active high
      mask Help: Output is active for one-cycle after each edge of the specified type (i.e. rising, falling, or both).  Latency is zero.
      mask TypeOptions edge: Rising | Falling | Both
      mask TypeOptions polarity: Active High | Active Low
      mask Display:
      | plot(x_in_num,0.5+y_in_num*0.2);
      | plot(x_out_num,0.5+y_out_num*0.2);
  out : Outport  VectorParamsAs1DForOutWhenUnconnected=off
  wires:
  posedge/1(out) -> Counter3/1
  in/1 -> posedge/1(in)
  Relational5/1 -> out/1, Counter3/2
  Constant5/1 -> Relational5/2
  Counter3/1 -> Relational5/1
